simulink model "MotorCtrl_FOC_Math"  (R2025b)
settings: Solver=FixedStepDiscrete  StartTime=0.0  StopTime=5  FixedStep=MC_Sim_BaseStep  RelTol=1e-3  EnableMultiTasking=on
values from neighbouring files (symbols this model uses):
  MC_ADC_BitNum = 0.0    [MotorControlDataDictionary_Math.sldd]
  MC_ADC_Offset = 0.0    [MotorControlDataDictionary_Math.sldd]
  MC_ADC_VRef = 1.0    [MotorControlDataDictionary_Math.sldd]
  MC_CSA_Gain = 1.0    [MotorControlDataDictionary_Math.sldd]
  MC_MOS_DeadTime = 1.3E-6    [MotorControlDataDictionary_Math.sldd]
  MC_Motor_Mechinal_Damp = 1.0E-5    [MotorControlDataDictionary_Math.sldd]
  MC_Motor_Mechinal_Fric = 0.0    [MotorControlDataDictionary_Math.sldd]
  MC_Motor_Mechinal_Inertia = 0.0103    [MotorControlDataDictionary_Math.sldd]
  MC_Motor_Phi = 0.0059190254913385806    [MotorControlDataDictionary_Math.sldd]
  MC_Motor_Rotor_Pn = 4.0    [MotorControlDataDictionary_Math.sldd]
  MC_Motor_Stator_Ld = 5.6345E-5    [MotorControlDataDictionary_Math.sldd]
  MC_Motor_Stator_Lq = 5.6345E-5    [MotorControlDataDictionary_Math.sldd]
  MC_Motor_Stator_Rs = 0.0286    [MotorControlDataDictionary_Math.sldd]
  MC_Param_CurrentPI_Ki = 0.0089705790612839825    [MotorControlDataDictionary_Math.sldd]
  MC_Param_CurrentPI_Kp = 0.283220860906427    [MotorControlDataDictionary_Math.sldd]
  MC_Param_CurrentPI_UdInteMax = 7.794228634059948    [MotorControlDataDictionary_Math.sldd]
  MC_Param_CurrentPI_UdInteMin = -7.794228634059948    [MotorControlDataDictionary_Math.sldd]
  MC_Param_CurrentPI_UdMax = 7.794228634059948    [MotorControlDataDictionary_Math.sldd]
  MC_Param_CurrentPI_UdMin = -7.794228634059948    [MotorControlDataDictionary_Math.sldd]
  MC_Param_CurrentPI_UqInteMax = 7.794228634059948    [MotorControlDataDictionary_Math.sldd]
  MC_Param_CurrentPI_UqInteMin = -7.794228634059948    [MotorControlDataDictionary_Math.sldd]
  MC_Param_CurrentPI_UqMax = 7.794228634059948    [MotorControlDataDictionary_Math.sldd]
  MC_Param_CurrentPI_UqMin = -7.794228634059948    [MotorControlDataDictionary_Math.sldd]
  MC_Param_Flux_Gamma = 750000.0    [MotorControlDataDictionary_Math.sldd]
  MC_Param_Flux_Lalpha = 5.6345E-5    [MotorControlDataDictionary_Math.sldd]
  MC_Param_Flux_Lbeta = 5.6345E-5    [MotorControlDataDictionary_Math.sldd]
  MC_Param_Flux_Ralpha = 0.0286    [MotorControlDataDictionary_Math.sldd]
  MC_Param_Flux_Rbeta = 0.0286    [MotorControlDataDictionary_Math.sldd]
  MC_Param_Luen_BEMFalpha = -17747.803709290976    [MotorControlDataDictionary_Math.sldd]
  MC_Param_Luen_BEMFbeta = -17747.803709290976    [MotorControlDataDictionary_Math.sldd]
  MC_Param_Luen_BEMFErr = 10.0    [MotorControlDataDictionary_Math.sldd]
  MC_Param_Luen_Currentalpha = -507.58718608572195    [MotorControlDataDictionary_Math.sldd]
  MC_Param_Luen_Currentbeta = -507.58718608572195    [MotorControlDataDictionary_Math.sldd]
  MC_Param_Luen_CurrentErr = 400.0    [MotorControlDataDictionary_Math.sldd]
  MC_Param_Luen_PLL_Ki = 0.24634532585119037    [MotorControlDataDictionary_Math.sldd]
  MC_Param_Luen_PLL_Kp = 125.66370614359172    [MotorControlDataDictionary_Math.sldd]
  MC_Param_Luen_Voltagealpha = 17747.803709290976    [MotorControlDataDictionary_Math.sldd]
  MC_Param_Luen_Voltagebeta = 17747.803709290976    [MotorControlDataDictionary_Math.sldd]
  MC_Param_PhasetoReal = 500.0    [MotorControlDataDictionary_Math.sldd]
  MC_Param_SMO_CoffA = 0.968326559588251    [MotorControlDataDictionary_Math.sldd]
  MC_Param_SMO_CoffB = 1.1074629514597569    [MotorControlDataDictionary_Math.sldd]
  MC_Param_SpeedCtrl_IdMax = 60.0    [MotorControlDataDictionary_Math.sldd]
  MC_Param_SpeedCtrl_IdMin = -60.0    [MotorControlDataDictionary_Math.sldd]
  MC_Param_SpeedCtrl_IqMax = 60.0    [MotorControlDataDictionary_Math.sldd]
  MC_Param_SpeedCtrl_IqMin = -60.0    [MotorControlDataDictionary_Math.sldd]
  MC_Param_SpeedPI_Ki = 0.57157085739428382    [MotorControlDataDictionary_Math.sldd]
  MC_Param_SpeedPI_Kp = 9.1114109857344836    [MotorControlDataDictionary_Math.sldd]
  MC_Param_SpeedtoTheta = 6.24E-5    [MotorControlDataDictionary_Math.sldd]
  MC_Param_SVPWM_DutyMax = 0.98    [MotorControlDataDictionary_Math.sldd]
  MC_Param_SVPWM_DutyMin = 0.02    [MotorControlDataDictionary_Math.sldd]
  MC_Param_SVPWM_SampleOffset1 = 0.02    [MotorControlDataDictionary_Math.sldd]
  MC_Param_SVPWM_SampleOffset2 = 0.015    [MotorControlDataDictionary_Math.sldd]
  MC_Param_SVPWM_SampleValid = 0.0096153846153846159    [MotorControlDataDictionary_Math.sldd]
  MC_Param_Zero = 0.0    [MotorControlDataDictionary_Math.sldd]
  MC_Sample_CurrentNoise = 1.0E-15    [MotorControlDataDictionary_Math.sldd]
  MC_Sample_Rs = 0.002    [MotorControlDataDictionary_Math.sldd]
  MC_Sample_VbusNoise = 1.0E-15    [MotorControlDataDictionary_Math.sldd]
  MC_Sim_BaseStep = 2.08E-8    [MotorControlDataDictionary_Math.sldd]
  MC_Sim_HFTStep = 6.24E-5    [MotorControlDataDictionary_Math.sldd]
  MC_Sim_MFTStep = 0.0019968    [MotorControlDataDictionary_Math.sldd]
libraries: simulink x28, nesl_utility x19, fl_lib x14, ee_lib x13, autolibpmsminterior x2, autolibinverter x1
(part 1 of 8)
settings Model: DataDictionary=MotorControlDataDictionary_Math.sldd  SimulationMode=accelerator  Creator=YXuan  LastModifiedBy=YXuan
settings SolverCC: AutoInsertRateTranBlk=on
settings OptimizationCC: DefaultParameterBehavior=Inlined  DefaultUnderspecifiedDataType=single  EnhancedBackFolding=on  PassReuseOutputArgsAs=Individual arguments  ZeroExternalMemoryAtStartup=off  ZeroInternalMemoryAtStartup=off  EfficientFloat2IntCast=on  OptimizeBlockOrder=speed  DifferentSizesBufferReuse=on  OptimizationCustomize=off  EfficientTunableParamExpr=on
settings DebuggingCC: ParameterPrecisionLossMsg=none
settings ModelReferenceCC: EnableRefExpFcnMdlSchedulingChecks=on
settings SFSimCC: MATLABDynamicMemAlloc=off
settings RTWCC: SystemTargetFile=ert.tlc  GenCodeOnly=on  TemplateMakefile=ert_default_tmf  Toolchain=Microsoft Visual C++ 2022 v17.0 | nmake (64-bit Windows)  GPUComputeCapability=3.5  Description=Embedded Coder
settings CodeAppCC: ForceParamTrailComments=on  IgnoreCustomStorageClasses=off  IgnoreTestpoints=on  OperatorAnnotations=on  SimulinkDataObjDesc=on  SFDataObjDesc=on  InsertBlockDesc=on
settings ERTTargetCC: ERTCustomFileTemplate=example_file_process.tlc  DynamicArrayContainerType=coder::array  TargetLangStandard=C99 (ISO)  InferredTypesCompatibility=on  GenerateSampleERTMain=on  CombineSignalStateStructs=on  SupportAbsoluteTime=off  SupportNonFinite=off  SupportComplex=off  RemoveDisableFunc=on

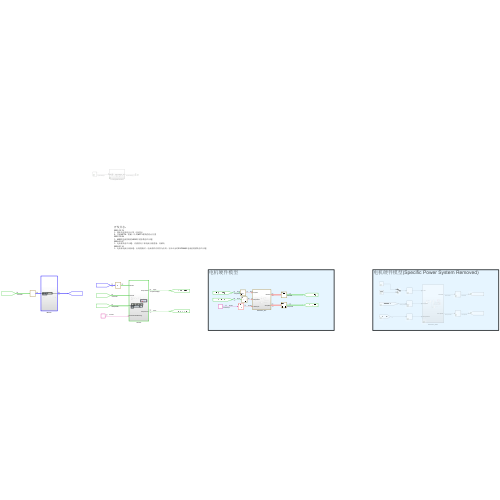
[thumbnail: Simulink's stored preview of the top-level diagram]
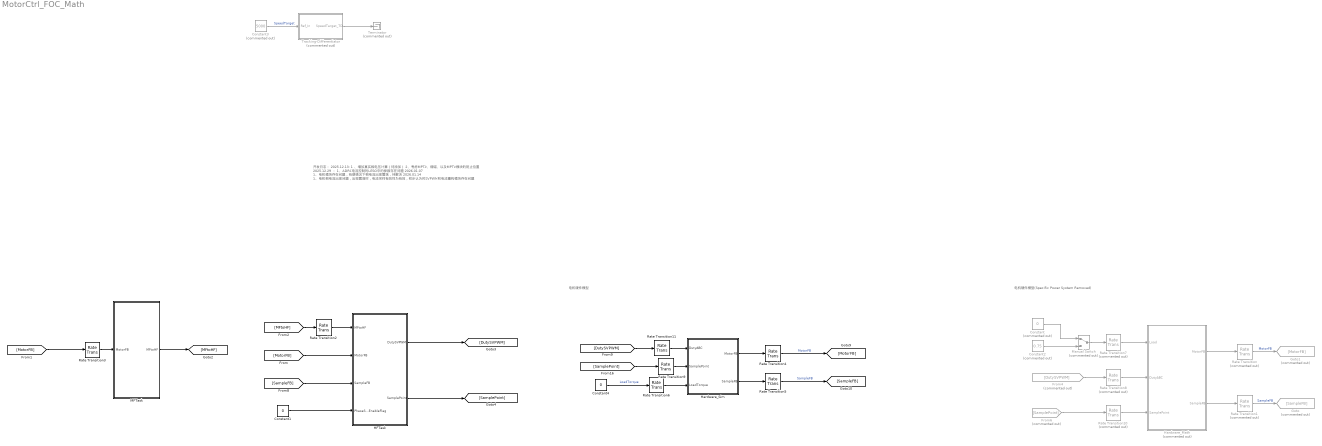
== system MotorCtrl_FOC_Math ==
  note: 电机硬件模型(Specific Power System Removed)
  note: 开发日志：
      | 2025.12.13:
      | 1、增加真实相电压计算（待添加）
      | 2、考虑MPTA、弱磁、以及MPTV模块的防止位置
      | 2025.12.29：
      | 1、ADRC电流控制的LESO中的参数存在问题
      | 2026.01.07
      | 1、电机模块存在问题，有感情况下相电流出现震荡，待解决
      | 2026.01.14
      | 1、电机相电流出现问题，出现震荡时，电流采样有效性为有效，初步认为时SVPWM和电流重构模块存在问题
  note: 电机硬件模型
  Constant : Constant  Commented=on  Value=0
  Constant1 : Constant  Value=0  OutDataTypeStr=boolean
  Constant2 : Constant  Commented=on  Value=0.75
  Constant3 : Constant  Commented=on  Value=5000  OutDataTypeStr=single
  Constant4 : Constant  Value=0
  From4 : From  Commented=on  GotoTag=DutySVPWM
  From6 : From  Commented=on  GotoTag=SamplePoint
  Goto : Goto  Commented=on  GotoTag=SampleFB
  Goto1 : Goto  Commented=on  GotoTag=MotorFB
  HFTask : Subsystem  TreatAsAtomicUnit=on  SystemSampleTime=MC_Sim_HFTStep
  Hardware_Math : Subsystem  Commented=on  SystemSampleTime=MC_Sim_BaseStep  VariantControl=MC_Hardware_Motor_Model ==1&MC_Hardware_MotorMOS_Model==1
  Hardware_Sim : Subsystem
  MFTask : Subsystem  TreatAsAtomicUnit=on  SystemSampleTime=MC_Sim_MFTStep
  Manual Switch : ManualSwitch  Commented=on
  Rate Transition : RateTransition  Commented=on  OutPortSampleTime=MC_Sim_HFTStep
  Rate Transition1 : RateTransition  Commented=on  OutPortSampleTime=MC_Sim_HFTStep
  Rate Transition10 : RateTransition  Commented=on  OutPortSampleTime=MC_Sim_BaseStep
  Rate Transition11 : RateTransition  OutPortSampleTime=MC_Sim_BaseStep
  Rate Transition2 : RateTransition  OutPortSampleTime=MC_Sim_HFTStep
  Rate Transition3 : RateTransition  OutPortSampleTime=MC_Sim_MFTStep
  Rate Transition4 : RateTransition  OutPortSampleTime=MC_Sim_HFTStep
  Rate Transition5 : RateTransition  OutPortSampleTime=MC_Sim_HFTStep
  Rate Transition6 : RateTransition  OutPortSampleTime=MC_Sim_BaseStep
  Rate Transition7 : RateTransition  Commented=on  OutPortSampleTime=MC_Sim_BaseStep
  Rate Transition8 : RateTransition  Commented=on  OutPortSampleTime=MC_Sim_BaseStep
  Rate Transition9 : RateTransition  OutPortSampleTime=MC_Sim_BaseStep
  Terminator : Terminator  Commented=on
  Tracking-Differentiator : Subsystem  Commented=on
  wires:
  Hardware_Math/2(SampleFB) -> Rate Transition1/1
  Rate Transition8/1 -> Hardware_Math/2(DutyABC)
  Hardware_Math/1(MotorFB) -> Rate Transition/1
  From6/1 -> Rate Transition10/1
  From4/1 -> Rate Transition8/1
  Rate Transition1/1 -> Goto/1  "SampleFB"
  Rate Transition10/1 -> Hardware_Math/3(SamplePoint)
  Rate Transition7/1 -> Hardware_Math/1(Load)
  Rate Transition/1 -> Goto1/1  "MotorFB"
  [MotorFB] -> Rate Transition3/1
  MFTask/1(MFtoHF) -> [MFtoHF]
  [MFtoHF] -> Rate Transition2/1
  Constant1/1 -> HFTask/4(PhaseShortEnableFlag)
  [SampleFB] -> HFTask/3(SampleFB)
  [MotorFB] -> HFTask/2(MotorFB)
  HFTask/1(DutySVPWM) -> [DutySVPWM]
  HFTask/2(SamplePoint) -> [SamplePoint]
  Rate Transition2/1 -> HFTask/1(MFtoHF)
  Rate Transition3/1 -> MFTask/1(MotorFB)
  Manual Switch/1 -> Rate Transition7/1
  Constant/1 -> Manual Switch/1
  Constant2/1 -> Manual Switch/2
  Tracking-Differentiator/1(SpeedTarget_TD) -> Terminator/1
  Constant3/1 -> Tracking-Differentiator/1(Ref_In)  "SpeedTarget"
  [DutySVPWM] -> Rate Transition11/1
  [SamplePoint] -> Rate Transition9/1
  Constant4/1 -> Rate Transition6/1  "LoadTorque"
  Hardware_Sim/1(MotorFB) -> Rate Transition4/1
  Hardware_Sim/2(SampleFB) -> Rate Transition5/1
  Rate Transition4/1 -> [MotorFB]  "MotorFB"
  Rate Transition5/1 -> [SampleFB]  "SampleFB"
  Rate Transition6/1 -> Hardware_Sim/3(LoadTorque)
  Rate Transition9/1 -> Hardware_Sim/2(SamplePoint)
  Rate Transition11/1 -> Hardware_Sim/1(DutyABC)

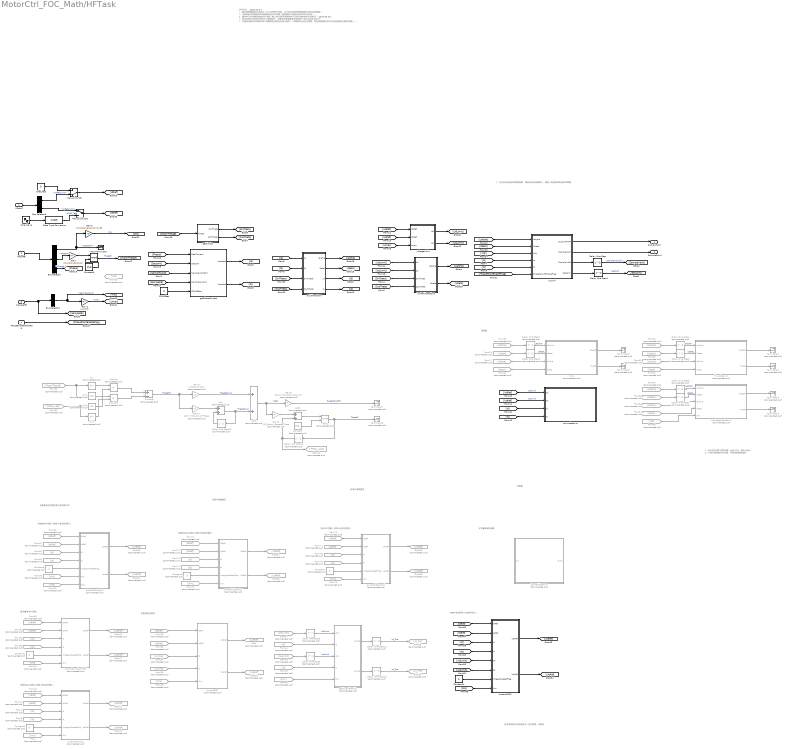
== system MotorCtrl_FOC_Math/HFTask ==
  note: 待更新电压控制的积分抗饱和方式
  note: 传统电流PI控制（前馈+电流抗饱和）
  note: 1、PLL存在问题(带宽问题，10hz可以，50hz溢出)
      | 2、方程反馈参数存在问题，导致观测角度超前
  note: 观测器
  note: 无差拍电流控制
  note: 开发日志：
      | 2025.03.24:
      | 1、磁链观测器增益应该适中（过小会导致不收敛，过大则会导致观测角度相位超前实际角度）
      | 2、无差拍电流控制是否采用预测电流进行控制？是否要进行旋转反电势的电压补偿？
      | 3、静态电压补偿模型增益如何设置？输入电压是采用理想电压还是采样的电机实际电压？
      | 2025.03.25:
      | 1、测试发现电压和电流呈现2个周期延时，无差拍应考虑做电流预测两个节拍
      | 2025.03.27：
      | 1、无差拍控制应采用延时两个周期的电流和电压进行延时一个周期的电流进行预测，然后用预测电流作为电流控制的反馈电流输入。
      | 2025.12.13:
      | 1、增加真实相电压计算（待添加）
      | 2、考虑MPTA、弱磁、以及MPTV模块的防止位置
      | 2026.01.01：
      | 1、增加卡尔曼滤波模块（未构建）
      | 2、增加PIR控制器（未整定参数）
      | 2026.01.28：
      | 1、发现ADRC的电流观测值初期收敛速度较慢，并且存在稳定的误差。
  note: 复矢量电流PI控制
  note: 传统电流PI控制（前馈+电压抗饱和）
  note: ADRC电流控制（性能待优化）
  note: 传统电流PID控制（前馈+电流抗饱和）
  note: 待进行参数整定
  note: 电流PIR控制（前馈+电流抗饱和）
  note: 待进行参数整定
  note: 卡尔曼滤波观测器
  note: 待构建
  note: 1、优化的单电阻采样移相策略、增加单边采样策略
      | 2、增加三电阻和两电阻采样策略
  note: 电流观测值与实际值存在一定的误差，待解决
  MFtoHF : Inport
  MotorFB : Inport  Port=2
  SampleFB : Inport  Port=3
  PhaseShortEnableFlag : Inport  Port=4
  Add : Sum  Commented=on
  Add1 : Sum  Commented=on
  Add2 : Sum  Commented=on
  Bus Selector : BusSelector  OutputSignals=SpeedM,ThetaM,PhaseI
  Bus Selector1 : BusSelector  OutputSignals=SampleVbus
  Bus Selector3 : BusSelector  OutputSignals=IdRefLimit,IqRefLimit
  CSAOffset : Constant  Value=0  OutDataTypeStr=single
  Constant : Constant  Commented=on  Value=2*pi  OutDataTypeStr=single
  Constant{1..3,5,7} (5 alike) : Constant  Commented=on  Value=0  OutDataTypeStr=boolean
  Constant4 : Constant  Value=0  OutDataTypeStr=boolean
  Constant6 : Constant  Value=2*pi  OutDataTypeStr=single
  Data Type Conversion : DataTypeConversion  OutDataTypeStr=single  RndMeth=Simplest  SaturateOnIntegerOverflow=off
  Delay One Step : Delay
  Delay One Step1 : Delay
  Delay One Step{8..11} (4 alike) : Delay  Commented=on  DelayLength=1
  Delay One Step12 : Delay  Commented=on  DelayLength=0
  Delay One Step13 : Delay  Commented=on  DelayLength=0
  Delay One Step{2..7} (6 alike) : Delay  Commented=on
  From{,39,46,59,70,75} (6 alike) : From  Commented=on  GotoTag=Wm
  From{10,35,50,60,71,76} (6 alike) : From  Commented=on  GotoTag=IdRef
  From{11,36,51,61,72,77} (6 alike) : From  Commented=on  GotoTag=IqRef
  From{2,44,52,62,73,78} (6 alike) : From  Commented=on  GotoTag=Id
  From25 : From  Commented=on  GotoTag=Ualpha
  From26 : From  Commented=on  GotoTag=Ubeta
  From27 : From  Commented=on  GotoTag=Ialpha
  From28 : From  Commented=on  GotoTag=Ibeta
  From{3,45,53,63,74,79} (6 alike) : From  Commented=on  GotoTag=Iq
  From31 : From  Commented=on  GotoTag=Ualpha
  From32 : From  Commented=on  GotoTag=Ubeta
  From33 : From  Commented=on  GotoTag=Ialpha
  From34 : From  Commented=on  GotoTag=Ibeta
  From37 : From  Commented=on  GotoTag=Id_Pre
  From38 : From  Commented=on  GotoTag=Iq_Pre
  From47 : From  Commented=on  GotoTag=UdLimit
  From48 : From  Commented=on  GotoTag=UqLimit
  From49 : From  Commented=on  GotoTag=We
  From54 : From  Commented=on  GotoTag=Ualpha
  From55 : From  Commented=on  GotoTag=Ubeta
  From56 : From  Commented=on  GotoTag=Ialpha
  From57 : From  Commented=on  GotoTag=Ibeta
  From58 : From  Commented=on  GotoTag=We
  From64 : From  Commented=on  GotoTag=Vdq
  From82 : From  Commented=on  GotoTag=Theta_Last
  From83 : From  Commented=on  GotoTag=MotorThetaE
  Gain : Gain  Gain=MC_Motor_Rotor_Pn  OutDataTypeStr=single
  Gain1 : Gain  Gain=1/sqrt(3)  OutDataTypeStr=single
  Gain2 : Gain  Gain=MC_Motor_Rotor_Pn*pi/30
  Gain3 : Gain  Commented=on  Gain=2*sqrt(2)/2*100
  Gain4 : Gain  Commented=on  Gain=100^2*MC_Sim_HFTStep
  Gain5 : Gain  Commented=on  Gain=MC_Param_SpeedtoTheta  OutDataTypeStr=single  RndMeth=Simplest
  Gain6 : Gain  Commented=on  Gain=30/(pi*MC_Motor_Rotor_Pn)  OutDataTypeStr=single  RndMeth=Simplest
  Goto{,14,30,32,37,39} (6 alike) : Goto  Commented=on  GotoTag=UdRef
  Goto{10,26..27,31,36,38} (6 alike) : Goto  Commented=on  GotoTag=UqRef
  Goto28 : Goto  Commented=on  GotoTag=Id_Pre
  Goto29 : Goto  Commented=on  GotoTag=Iq_Pre
  Goto33 : Goto  Commented=on  GotoTag=Vdq
  Goto40 : Goto  Commented=on  GotoTag=Theta_Last
  Idref_Test : Constant  Value=0  OutDataTypeStr=single
  LuenbergerObservor : Subsystem  Commented=on
  Manual Switch : ManualSwitch  CurrentSetting=0
  Manual Switch1 : ManualSwitch
  Mod : Math  Operator=mod
  Mod1 : Math  Commented=on  Operator=mod
  Product : Product  Commented=on
  Product1 : Product  Commented=on
  Sin : Trigonometry  Commented=on  OutputSignalType=real
  Sin1 : Trigonometry  Commented=on  Operator=cos  OutputSignalType=real
  Sin2 : Trigonometry  Commented=on  OutputSignalType=real
  Sin3 : Trigonometry  Commented=on  Operator=cos  OutputSignalType=real
  Sine Wave : Sin  Amplitude=20  Frequency=2*pi*1  SampleTime=MC_Sim_HFTStep
  Subtract : Sum  Commented=on  Inputs=+-
  Terminator : Terminator
  Terminator{1..8} (8 alike) : Terminator  Commented=on
  axisTransform : Subsystem
  currentADRC : Subsystem
  currentComplexPICtrl : Subsystem  Commented=on
  currentDBC : Subsystem  Commented=on
  currentPIControl : Subsystem  Commented=on
  currentPIControl1 : Subsystem  Commented=on
  currentPIDControl : Subsystem  Commented=on
  currentPIRControl : Subsystem  Commented=on
  fluxobservor : Subsystem  Commented=on
  getCurrentPredict : Subsystem  Commented=on
  getPhaseCurrent : Subsystem
  getSinCos : Subsystem
  invParkTransform : Subsystem
  karmalObservor : Subsystem  Commented=on
  scvmobservor : Subsystem
  smo : Subsystem  Commented=on
  svpwm : Subsystem  TreatAsAtomicUnit=on
  voltageLimit : Subsystem
  DutySVPWM : Outport
  SamplePoint : Outport  Port=2
  wires:
  MFtoHF/1 -> Bus Selector3/1
  Delay One Step2/1 -> smo/1(Valpha)  "Ualpha"
  From25/1 -> Delay One Step2/1
  Delay One Step3/1 -> smo/2(Vbeta)  "Ubeta"
  From26/1 -> Delay One Step3/1
  From27/1 -> smo/3(Ialpha)
  From28/1 -> smo/4(Ibeta)
  smo/1(Speed) -> Terminator2/1
  smo/2(Theta) -> Terminator3/1
  [PhaseShortEnableFlag] -> svpwm/6(PhaseShortEnableFlag)
  [Umax] -> voltageLimit/3(Umax)
  svpwm/4(SectorN) -> Delay One Step1/1
  axisTransform/2(Ibeta) -> [Ibeta]
  svpwm/3(SampleValid) -> Delay One Step/1
  svpwm/1(DutySVPWM) -> DutySVPWM/1
  [SampleFB] -> getPhaseCurrent/4(SampleCurrent)
  [SectorN] -> getPhaseCurrent/2(SectorN)
  [UdRef] -> voltageLimit/1(UdRef)
  [UdLimit] -> invParkTransform/1(Ud)
  currentPIControl/1(UdRef) -> Goto14/1
  [Ubeta] -> svpwm/2(Vbeta)
  axisTransform/1(Ialpha) -> [Ialpha]
  [UqRef] -> voltageLimit/2(UqRef)
  [Ualpha] -> svpwm/1(Valpha)
  [Ia] -> axisTransform/1(Ia)
  svpwm/2(SamplePoint) -> SamplePoint/1
  currentPIControl/2(UqRef) -> Goto10/1
  [Vdc] -> svpwm/3(Vdc)
  voltageLimit/1(Ud) -> [UdLimit]
  [MotorThetaE] -> getSinCos/1(Theta)
  From2/1 -> currentPIControl/3(Id)
  getSinCos/1(SinTheta) -> [SinTheta]
  [SampleValid] -> getPhaseCurrent/3(SampleValid[2])
  axisTransform/3(Id) -> [Id]
  getPhaseCurrent/2(Ibselect) -> [Ib]
  From/1 -> currentPIControl/6(Wm)
  axisTransform/4(Iq) -> [Iq]
  From3/1 -> currentPIControl/4(Iq)
  Constant2/1 -> currentPIControl/5(IntregralResetFlag)
  [Ib] -> axisTransform/2(Ib)
  [UqLimit] -> invParkTransform/2(Uq)
  [SinTheta] -> invParkTransform/3(SinTheta)
  Delay One Step1/1 -> [SectorN]  "SectorN"
  [CosTheta] -> invParkTransform/4(CosTheta)
  [PhaseI] -> getPhaseCurrent/1(RealCurrent)
  invParkTransform/1(Ualpha) -> [Ualpha]
  Delay One Step/1 -> [SampleValid]  "SampleValid[2]"
  getSinCos/2(CosTheta) -> [CosTheta]
  voltageLimit/2(Uq) -> [UqLimit]
  [SinTheta] -> axisTransform/3(SinTheta)
  getPhaseCurrent/1(Iaselect) -> [Ia]
  CSAOffset/1 -> getPhaseCurrent/5(CSAOffset)
  [CosTheta] -> axisTransform/4(CosTheta)
  invParkTransform/2(Ubeta) -> [Ubeta]
  [Ib] -> svpwm/5(Ib)
  [Ia] -> svpwm/4(Ia)
  Bus Selector/2 -> Gain/1  "<ThetaM>"
  PhaseShortEnableFlag/1 -> [PhaseShortEnableFlag]
  Bus Selector/1 -> Terminator/1, Gain2/1  "<SpeedM>"
  Mod/1 -> [MotorThetaE]  "ThetaE"
  Bus Selector/3 -> [PhaseI]  "<PhaseI>"
  Gain/1 -> Mod/1
  Bus Selector1/1 -> Gain1/1, [Vdc]  "<SampleVbus>"
  SampleFB/1 -> [SampleFB], Bus Selector1/1
  Gain1/1 -> [Umax]  "Umax"
  Constant6/1 -> Mod/2
  MotorFB/1 -> Bus Selector/1
  From10/1 -> currentPIControl/1(IdRef)
  From11/1 -> currentPIControl/2(IqRef)
  From34/1 -> fluxobservor/4(Ibeta)
  From33/1 -> fluxobservor/3(Ialpha)
  From32/1 -> Delay One Step5/1
  From31/1 -> Delay One Step4/1
  Delay One Step4/1 -> fluxobservor/1(Valpha)  "Ualpha"
  Delay One Step5/1 -> fluxobservor/2(Vbeta)  "Ubeta"
  fluxobservor/1(Speed) -> Terminator1/1
  fluxobservor/2(Theta) -> Terminator4/1
  currentDBC/2(UqRef) -> Goto26/1
  From36/1 -> currentDBC/2(IqRef)
  From35/1 -> currentDBC/1(IdRef)
  From37/1 -> currentDBC/3(Id)
  From38/1 -> currentDBC/4(Iq)
  From39/1 -> currentDBC/5(Wm)
  [UqRef] -> scvmobservor/2(Vq)  "UqLimit"
  [UdRef] -> scvmobservor/1(Vd)  "UdLimit"
  [Id] -> scvmobservor/3(Id)
  [Iq] -> scvmobservor/4(Iq)
  Gain2/1 -> [We]  "We"
  From44/1 -> getCurrentPredict/2(Id)
  From45/1 -> getCurrentPredict/4(Iq)
  From46/1 -> getCurrentPredict/5(Wm)
  From47/1 -> Delay One Step8/1
  From48/1 -> Delay One Step9/1
  getCurrentPredict/1(Id_Pre) -> Delay One Step12/1
  getCurrentPredict/2(Iq_Pre) -> Delay One Step13/1
  currentDBC/1(UdRef) -> Goto/1
  Delay One Step8/1 -> getCurrentPredict/1(Ud1)  "UdLimit"
  Delay One Step9/1 -> getCurrentPredict/3(Uq1)  "UqLimit"
  Delay One Step12/1 -> Goto28/1  "Id_Pre"
  Delay One Step13/1 -> Goto29/1  "Iq_Pre"
  From51/1 -> currentComplexPICtrl/2(IqRef)
  From50/1 -> currentComplexPICtrl/1(IdRef)
  Constant1/1 -> currentComplexPICtrl/5(IntregralResetFlag)
  From53/1 -> currentComplexPICtrl/4(Iq)
  From49/1 -> currentComplexPICtrl/6(Wm)
  From52/1 -> currentComplexPICtrl/3(Id)
  currentComplexPICtrl/2(UqRef) -> Goto27/1
  currentComplexPICtrl/1(UdRef) -> Goto30/1
  LuenbergerObservor/1(Speed) -> Terminator5/1
  LuenbergerObservor/2(Theta) -> Terminator6/1
  From57/1 -> LuenbergerObservor/4(Ibeta)
  From56/1 -> LuenbergerObservor/3(Ialpha)
  From55/1 -> Delay One Step7/1
  From54/1 -> Delay One Step6/1
  Delay One Step7/1 -> LuenbergerObservor/2(Vbeta)  "Ubeta"
  Delay One Step6/1 -> LuenbergerObservor/1(Valpha)  "Ualpha"
  From58/1 -> LuenbergerObservor/5(We)
  From61/1 -> currentPIControl1/2(IqRef)
  From60/1 -> currentPIControl1/1(IdRef)
  Constant3/1 -> currentPIControl1/5(IntregralResetFlag)
  From63/1 -> currentPIControl1/4(Iq)
  From59/1 -> currentPIControl1/6(Wm)
  From62/1 -> currentPIControl1/3(Id)
  currentPIControl1/2(UqRef) -> Goto31/1
  currentPIControl1/1(UdRef) -> Goto32/1
  From64/1 -> currentPIControl1/7(Vdq)
  currentADRC/1(UdRef) -> [UdRef]
  currentADRC/2(UqRef) -> [UqRef]
  [Id] -> currentADRC/3(Id)
  [We] -> currentADRC/8(Wm)
  [Iq] -> currentADRC/4(Iq)
  Constant4/1 -> currentADRC/7(IntregralResetFlag)
  [IdRef] -> currentADRC/1(IdRef)
  [IqRef] -> currentADRC/2(IqRef)
  Constant5/1 -> currentPIDControl/5(IntregralResetFlag)
  From71/1 -> currentPIDControl/1(IdRef)
  currentPIDControl/1(UdRef) -> Goto37/1
  From73/1 -> currentPIDControl/3(Id)
  From72/1 -> currentPIDControl/2(IqRef)
  currentPIDControl/2(UqRef) -> Goto36/1
  From70/1 -> currentPIDControl/6(Wm)
  From74/1 -> currentPIDControl/4(Iq)
  Bus Selector3/1 -> Manual Switch/2  "<IdRefLimit>"
  Bus Selector3/2 -> Manual Switch1/1  "<IqRefLimit>"
  Sine Wave/1 -> Data Type Conversion/1
  Manual Switch/1 -> [IdRef]
  Idref_Test/1 -> Manual Switch/1
  Manual Switch1/1 -> [IqRef]
  Data Type Conversion/1 -> Manual Switch1/2  "IqRef_Test"
  From79/1 -> currentPIRControl/4(Iq)
  From75/1 -> currentPIRControl/6(Wm)
  currentPIRControl/2(UqRef) -> Goto38/1
  From77/1 -> currentPIRControl/2(IqRef)
  From78/1 -> currentPIRControl/3(Id)
  currentPIRControl/1(UdRef) -> Goto39/1
  From76/1 -> currentPIRControl/1(IdRef)
  Constant7/1 -> currentPIRControl/5(IntregralResetFlag)
  [UdLimit] -> currentADRC/5(Ud)
  [UqLimit] -> currentADRC/6(Uq)
  Gain5/1 -> Add2/1
  Delay One Step10/1 -> Add/2
  Constant/1 -> Mod1/2
  Mod1/1 -> Terminator8/1, Delay One Step11/1  "ThetaPI"
  Delay One Step11/1 -> Goto40/1, Add2/2
  Gain3/1 -> Add1/1  "ThetaErr_Kp"
  Add1/1 -> Gain6/1, Gain5/1  "WePI"
  Add2/1 -> Mod1/1
  Gain6/1 -> Terminator7/1  "SpeedPI_RPM"
  Subtract/1 -> Gain3/1, Gain4/1  "ThetaErr"
  Add/1 -> Add1/2, Delay One Step10/1  "ThetaErr_Ki"
  Gain4/1 -> Add/1
  From83/1 -> Sin1/1, Sin/1
  From82/1 -> Sin2/1, Sin3/1
  Sin/1 -> Product/1
  Sin3/1 -> Product/2
  Product/1 -> Subtract/1
  Sin1/1 -> Product1/1
  Sin2/1 -> Product1/2
  Product1/1 -> Subtract/2

== system MotorCtrl_FOC_Math/Hardware_Math ==
  Load : Inport
  DutyABC : Inport  Port=2
  SamplePoint : Inport  Port=3
  Add : Sum
  Add1 : Sum
  Add2 : Sum
  AngleProcess : Subsystem
  Band-Limited White Noise : simulink/Sources/Band-Limited White Noise  Cov=[MC_Sample_CurrentNoise]  Ts=MC_Sim_BaseStep  seed=[23341]
  Band-Limited White Noise1 : simulink/Sources/Band-Limited White Noise  Cov=[MC_Sample_VbusNoise]  Ts=MC_Sim_BaseStep  seed=[23341]
  Bus Creator : BusCreator  Inputs=5
  Bus Creator1 : BusCreator  Inputs=2
  Bus Selector : BusSelector  OutputSignals=Te,Wm,ThetaM
  Data Type Conversion{,1..3} (4 alike) : DataTypeConversion  OutDataTypeStr=single  SaturateOnIntegerOverflow=off  RndMeth=Floor
  Data Type Conversion4 : DataTypeConversion  Commented=on  OutDataTypeStr=single  SaturateOnIntegerOverflow=off  RndMeth=Floor
  Data Type Conversion5 : DataTypeConversion  Commented=on  OutDataTypeStr=single  SaturateOnIntegerOverflow=off  RndMeth=Floor
  From5 : From  Commented=on  GotoTag=Idq
  From6 : From  Commented=on  GotoTag=Vdq
  Gain : Gain  Gain=0.00000154
  Gain1 : Gain  Gain=30/pi
  Goto5 : Goto  Commented=on  GotoTag=Hall
  Goto6 : Goto  Commented=on  GotoTag=Vdq
  Goto7 : Goto  Commented=on  GotoTag=Idq
  MotorHardware : Subsystem
  Mux : Mux  Commented=on  Inputs=3
  Mux1 : Mux  Commented=on  Inputs=2
  Mux2 : Mux  Commented=on  Inputs=2
  PWMGenerate : Subsystem  SystemSampleTime=MC_Sim_BaseStep
  Square : Math  Operator=square
  VbusSample : Subsystem
  currentSample : Subsystem  Variant=on  VariantControl=Subsystem
  MotorFB : Outport
  SampleFB : Outport  Port=2
  wires:
  Band-Limited White Noise/1 -> Add/2
  Add/1 -> currentSample/2(Current)
  Add1/1 -> VbusSample/1(Vbus)
  Band-Limited White Noise1/1 -> Add1/2
  [CurrentSampleTrigger] -> currentSample/1(SampleTrigger)
  PWMGenerate/2(CurrentSamplTrigger) -> [CurrentSampleTrigger]
  DutyABC/1 -> PWMGenerate/1(DutyABC)
  SamplePoint/1 -> PWMGenerate/2(SamplePoint)
  Load/1 -> [Load_Input]
  Gain1/1 -> [Wm], Data Type Conversion/1
  AngleProcess/1(Out1) -> Bus Creator/1
  [PhaseV] -> Data Type Conversion2/1
  [PhaseI] -> Data Type Conversion3/1
  VbusSample/1(VbusSample) -> Bus Creator1/1  "SampleVus"
  currentSample/1(SampleCurrent) -> Bus Creator1/2
  Bus Creator1/1 -> SampleFB/1  "SampleFB"
  PWMGenerate/1(Gate) -> MotorHardware/2(PWM)  "PWM"
  MotorHardware/1(Vabc) -> [PhaseV]
  MotorHardware/2(Iabc) -> [PhaseI]
  MotorHardware/3(m) -> Bus Selector/1
  MotorHardware/5(Current) -> Add/1
  MotorHardware/4(Vbus) -> Add1/1
  Data Type Conversion/1 -> Bus Creator/2  "SpeedM"
  Data Type Conversion1/1 -> Bus Creator/3  "Te"
  Data Type Conversion2/1 -> Bus Creator/4  "PhaseV"
  Data Type Conversion3/1 -> Bus Creator/5  "PhaseI"
  Bus Creator/1 -> MotorFB/1  "MotorFB"
  Add2/1 -> MotorHardware/1(mec)
  [Load_Input] -> Add2/2
  [Wm] -> Square/1
  Gain/1 -> Add2/1
  ? -> Mux/1  "<Hall effect signal h_a>"
  ? -> Mux/2  "<Hall effect signal h_b>"
  ? -> Mux/3  "<Hall effect signal h_c>"
  Mux/1 -> Goto5/1  "MotorHall"
  Mux1/1 -> Goto6/1  "Vdq"
  ? -> Mux1/2  "<Stator voltage Vs_q (V)>"
  ? -> Mux1/1  "<Stator voltage Vs_d (V)>"
  ? -> Mux2/1  "<Stator current is_d (A)>"
  ? -> Mux2/2  "<Stator current is_q (A)>"
  Mux2/1 -> Goto7/1  "Idq"
  From6/1 -> Data Type Conversion4/1
  From5/1 -> Data Type Conversion5/1
  Data Type Conversion5/1 -> ?  "Idq"
  Data Type Conversion4/1 -> ?  "Vdq"
  Square/1 -> Gain/1
  Bus Selector/2 -> Gain1/1  "<Wm>"
  Bus Selector/3 -> AngleProcess/1(In1)  "<ThetaM>"
  Bus Selector/1 -> Data Type Conversion1/1  "<Te>"

== system MotorCtrl_FOC_Math/Hardware_Sim ==
  DutyABC : Inport
  SamplePoint : Inport  Port=2
  LoadTorque : Inport  Port=3
  Abs : Abs  SaturateOnIntegerOverflow=off
  Add : Sum
  Add1 : Sum
  AngleProcess : Subsystem
  Band-Limited White Noise : simulink/Sources/Band-Limited White Noise  Cov=[MC_Sample_CurrentNoise]  Ts=MC_Sim_BaseStep  seed=[23341]
  Band-Limited White Noise1 : simulink/Sources/Band-Limited White Noise  Cov=[MC_Sample_VbusNoise]  Ts=MC_Sim_BaseStep  seed=[23341]
  Bus Creator : BusCreator  Inputs=3
  Bus Creator1 : BusCreator  Inputs=2
  Bus Selector : BusSelector  OutputSignals=MtrTrq,MtrPos,VdSync,VqSync,IqSync,IdSync
  Constant5 : Constant  Value=13.5
  Data Type Conversion1 : DataTypeConversion  OutDataTypeStr=single  RndMeth=Simplest  SaturateOnIntegerOverflow=off
  Data Type Conversion2 : DataTypeConversion  OutDataTypeStr=single  RndMeth=Simplest  SaturateOnIntegerOverflow=off
  Data Type Conversion3 : DataTypeConversion  OutDataTypeStr=single  RndMeth=Simplest  SaturateOnIntegerOverflow=off
  Delay One Step : Delay  DelayLength=1
  Delay One Step1 : Delay  DelayLength=1
  Delay One Step2 : Delay  DelayLength=1
  Interior PMSM : autolibpmsminterior/Interior PMSM  port_config=Torque  sim_type=Discrete  Ts=MC_Sim_BaseStep  P=MC_Motor_Rotor_Pn  Rs=MC_Motor_Stator_Rs  Ldq=[MC_Motor_Stator_Ld MC_Motor_Stator_Lq]  KConstText=Permanent flux linkage constant (lambda_pm):  lambda_pm=MC_Motor_Phi  Ke=159.9771  mechanical=[MC_Motor_Mechinal_Inertia,MC_Motor_Mechinal_Damp,MC_Motor_Mechinal_Fric]  idq0=[0 0]  theta_init=0  omega_init=0  KConst=0.2205  lambda_pm_calc=0.2205  Kt=0.07  RefBlkName='autolibpmsminterior/Interior PMSM'  aMode=5
      settings: LibrarySourceBlock=mcblib/Electrical Systems/Motors/Interior PMSM
  Manual Switch : ManualSwitch
  PWMGenerate : Subsystem  SystemSampleTime=MC_Sim_BaseStep
  Sine Wave : Sin  Amplitude=13.5*sqrt(2)  Frequency=50*2*pi
  Terminator2 : Terminator
  Three-Phase Voltage Source Inverter : autolibinverter/Three-Phase Voltage Source Inverter  InvrtrTmpInpEnbl=off  enable_hdl=off  model_type=Switch inputs  fs=10000  w_eff_bp=[-1000 -500 0 500 1000]  n1=128  T_eff_bp=[-200 -100 0 100 200]  Temp_eff_bp=[213.15 293.15 373.15]  n2=128  ploss_table=[1 0.999 0.989 0.997 0.996;0.995 0.994 0.993 0.992 0.991;0.990 0.989 0.988 0.987 0.986;0.985 0.984 0.983 0.982 0.981;0.980 0.979 0.978 0.977 0.976]  ploss_table_3d=cat(3,0.95*[1 0.999 0.989 0.997 0.996;0.995 0.994 0.993 0.992 0.991;0.990 0.989 0.988 0.987 0.986;0.985 0.984 0.983 0.982 0.981;0.980 0.979 0.978 0.977 0.976],[1 0.999 0.989 0.997 0.996;0.995 0.994 0.993 0.992 0.991;0.990 0.989 0.988 0.987 0.986;0.985 0.984 0.983 0.982 0.981;0.980 0.979 0.978 0.977 0.976],0.92*[1 0.999 0.989 0.997 0.996;0.995 0.994 0.993 0.992 0.991;0.990 0.989 0.988 0.987 0.986;0.985 0.984 0.983 0.982 0.981;0.980 0.979 0.978 0.977 0.976])  preExtrapFlag=off  u1max=1000  u1min=-1000  u2max=200  u2min=-200  intPrec=23  RefBlkName='autolibmappedmotor/Mapped Motor'  CalLossMapData={}  CalLossWithTempMapData={}
      settings: LibrarySourceBlock=autolibemachines/Three-Phase Voltage Source Inverter
  VbusSample : Subsystem
  currentSample : Subsystem  Variant=on  VariantControl=Subsystem
  MotorFB : Outport
  SampleFB : Outport  Port=2
  wires:
  Data Type Conversion2/1 -> Bus Creator/2  "SpeedM"
  [Vbus] -> Three-Phase Voltage Source Inverter/2
  [BusCurr] -> Add/1
  Delay One Step2/1 -> Three-Phase Voltage Source Inverter/3
  [GateDrive] -> Three-Phase Voltage Source Inverter/1
  Interior PMSM/1 -> Bus Selector/1  "Motor_Info"
  Bus Selector/1 -> [MtrTrq]  "<MtrTrq>"
  Delay One Step1/1 -> Three-Phase Voltage Source Inverter/5
  Interior PMSM/3 -> [MtrSpd]  "SpeedM"
  [PhaseCurr] -> Delay One Step2/1
  Three-Phase Voltage Source Inverter/2 -> Interior PMSM/2  "PhaseVoltage"
  Interior PMSM/2 -> [PhaseCurr]  "PhaseI"
  [MtrSpd] -> Data Type Conversion2/1
  [Vbus] -> Add1/1
  Bus Creator1/1 -> SampleFB/1
  SamplePoint/1 -> PWMGenerate/2(SamplePoint)
  [PhaseCurr] -> Data Type Conversion1/1
  Three-Phase Voltage Source Inverter/1 -> Terminator2/1  "Inverter_Info"
  Delay One Step/1 -> Three-Phase Voltage Source Inverter/4
  Add/1 -> currentSample/2(Current)
  Data Type Conversion3/1 -> Bus Creator/1  "ThetaM"
  VbusSample/1(VbusSample) -> Bus Creator1/1  "SampleVbus"
  PWMGenerate/1(Gate) -> [GateDrive]  "PWM"
  Bus Selector/2 -> [MtrPos]  "<MtrPos>"
  [MtrPos] -> AngleProcess/1(In1)
  [MtrTrq] -> Delay One Step/1
  Data Type Conversion1/1 -> Bus Creator/3  "PhaseI"
  AngleProcess/1(Out1) -> Data Type Conversion3/1
  Three-Phase Voltage Source Inverter/3 -> [BusCurr]  "BusCurr"
  [CurrentSampleTrigger] -> currentSample/1(SampleTrigger)
  [MtrSpd] -> Delay One Step1/1
  PWMGenerate/2(CurrentSamplTrigger) -> [CurrentSampleTrigger]
  Add1/1 -> VbusSample/1(Vbus)
  LoadTorque/1 -> Interior PMSM/1
  Band-Limited White Noise/1 -> Add/2
  Band-Limited White Noise1/1 -> Add1/2
  currentSample/1(SampleCurrent) -> Bus Creator1/2
  Bus Creator/1 -> MotorFB/1
  DutyABC/1 -> PWMGenerate/1(DutyABC)
  Sine Wave/1 -> Abs/1
  Constant5/1 -> Manual Switch/1  "SampleVbus"
  Manual Switch/1 -> [Vbus]  "SampleVbus"
  Abs/1 -> Manual Switch/2  "SampleVbus"
  Bus Selector/3 -> [VdSync]  "<VdSync>"
  Bus Selector/6 -> [IdSync]  "<IdSync>"
  Bus Selector/5 -> [IqSync]  "<IqSync>"
  Bus Selector/4 -> [VqSync]  "<VqSync>"

== system MotorCtrl_FOC_Math/MFTask ==
  note: ADRC转速控制器
  note: PI转速控制器
  note: 滑膜转速控制器
  note: 开发日志：
      | 2025.11.03:
      | 1、初步完成ADRC控制架构，微分跟踪器存在问题，待调试
      | 2026.01.05：
      | 1、电流环ADRC的最速微分跟踪器存在问题，LESO和NLESF存在参数问题，待优化
      | 2026.01.28：
      | 1、仿真发现转速pi控制器200rpm是存在先维持在205rpm一段时间，然后突然调整至200rpm，造成参考电流突变。
      | 2、滑膜控制器200rpm会稳定在199rpm左右，并有微弱上升趋势
  note: 1、TD待优化
      | 2、LESO待参数优化
      | 3、NFLESS待参数优化
  MotorFB : Inport
  Bus Creator : BusCreator  Inputs=2
  Bus Selector : BusSelector  OutputSignals=SpeedM
  Constant : Constant  Value=1000  OutDataTypeStr=single
  Constant1 : Constant  Commented=on  Value=40  OutDataTypeStr=single
  Constant2 : Constant  Commented=on  Value=0  OutDataTypeStr=single
  From6 : From  Commented=on  GotoTag=SpeedTarget
  From7 : From  Commented=on  GotoTag=SpeedMotor
  From8 : From  Commented=on  GotoTag=SpeedTarget
  From9 : From  Commented=on  GotoTag=SpeedMotor
  Goto10 : Goto  Commented=on  GotoTag=IdRef
  Goto11 : Goto  Commented=on  GotoTag=IqRef
  Goto2 : Goto  Commented=on  GotoTag=IdRef
  Goto3 : Goto  Commented=on  GotoTag=IqRef
  Goto8 : Goto  Commented=on  GotoTag=IdRef
  Goto9 : Goto  Commented=on  GotoTag=IqRef
  adrcofSpeed : Subsystem  Commented=on
  getCurrentLimit : Subsystem
  piofSpeed : Subsystem  Commented=on
  smcofSpeed : Subsystem
  MFtoHF : Outport
  wires:
  MotorFB/1 -> Bus Selector/1
  Bus Selector/1 -> [SpeedMotor]  "<SpeedM>"
  Bus Creator/1 -> MFtoHF/1
  smcofSpeed/1(IdRef) -> [IdRef]
  smcofSpeed/2(IqRef) -> [IqRef]
  piofSpeed/1(IdRef) -> Goto2/1
  piofSpeed/2(IqRef) -> Goto3/1
  getCurrentLimit/2(IqRefLimit) -> [IqRefLimit]
  getCurrentLimit/1(IdRefLimit) -> [IdRefLimit]
  [IdRefLimit] -> Bus Creator/1
  [IqRefLimit] -> Bus Creator/2
  [SpeedTarget] -> smcofSpeed/1(SpeedTarget)
  [SpeedMotor] -> smcofSpeed/2(SpeedReal)
  [IdRef] -> getCurrentLimit/1(IdRef)
  [IqRef] -> getCurrentLimit/2(IqRef)
  From6/1 -> piofSpeed/1(SpeedTarget)
  From7/1 -> piofSpeed/2(SpeedReal)
  Constant/1 -> [SpeedTarget]  "SpeedTarget"
  adrcofSpeed/2(IqRef) -> Goto9/1
  adrcofSpeed/1(IdRef) -> Goto8/1
  From9/1 -> adrcofSpeed/2(SpeedReal)
  From8/1 -> adrcofSpeed/1(SpeedTarget)
  Constant1/1 -> Goto11/1
  Constant2/1 -> Goto10/1
